simulink model "hybrid_model"  (R2021a)
settings: Solver=ode4  StartTime=0.0  StopTime=TMax  FixedStep=DT  MaxStep=DT  RelTol=1e-3  EnableMultiTasking=on
undefined symbols (not defined in the file or in its folder): OutList, strmatch
settings Model: Creator=bjonkman  LastModifiedBy=cam
settings SolverCC: AlgebraicLoopSolver=TrustRegion
settings DataIOCC: LimitDataPoints=on  SaveFormat=Array  SaveOutput=off  SaveTime=off  ReturnWorkspaceOutputs=off  SignalLoggingName=sigsOut
settings OptimizationCC: ExpressionDepthLimit=2147483647  LifeSpan=inf
settings DebuggingCC: SaveWithParameterizedLinksMsg=none  UnderspecifiedInitializationDetection=Classic  MergeDetectMultiDrivingBlocksExec=none  SignalResolutionControl=TryResolveAllWithWarning  InheritedTsInSrcMsg=none  MultiTaskDSMMsg=warning  MultiTaskCondExecSysMsg=none  FcnCallInpInsideContextMsg=warning  StateNameClashWarn=warning  SFUnexpectedBacktrackingDiag=warning  SFNoUnconditionalDefaultTransitionDiag=warning  SFExecutionAtInitializationDiag=none  SFMachineParentedDataDiag=warning  ArithmeticOperatorsInVariantConditions=warning
settings HardwareCC: ProdBitPerPointer=32  ProdBitPerSizeT=32  ProdBitPerPtrDiffT=32  ProdLargestAtomicFloat=None  ProdIntDivRoundTo=Undefined  ProdEndianess=Unspecified  ProdWordSize=32  ProdHWDeviceType=32-bit Generic  TargetBitPerLong=64  TargetBitPerPointer=64  TargetBitPerSizeT=64  TargetBitPerPtrDiffT=64  TargetLongLongMode=on  TargetIntDivRoundTo=Zero  TargetEndianess=LittleEndian  TargetWordSize=64  TargetHWDeviceType=MATLAB Host  ProdEqTarget=off
settings ModelReferenceCC: PropagateSignalLabelsOutOfModel=off
settings SFSimCC: SimUseLocalCustomCode=off  CustomCodeUndefinedFunction=UseInterfaceOnly
settings RTWCC: RTWUseLocalCustomCode=off
settings CodeAppCC: StateflowObjectComments=on
settings GRTTargetCC: TargetLangStandard=C89/C90 (ANSI)  CombineOutputUpdateFcns=off  GRTInterface=on
settings ConfigComp: CovMetricSettings=dw  CovSaveCumulativeToWorkspaceVar=on  CovSaveSingleToWorkspaceVar=on  CovExternalEMLEnable=off

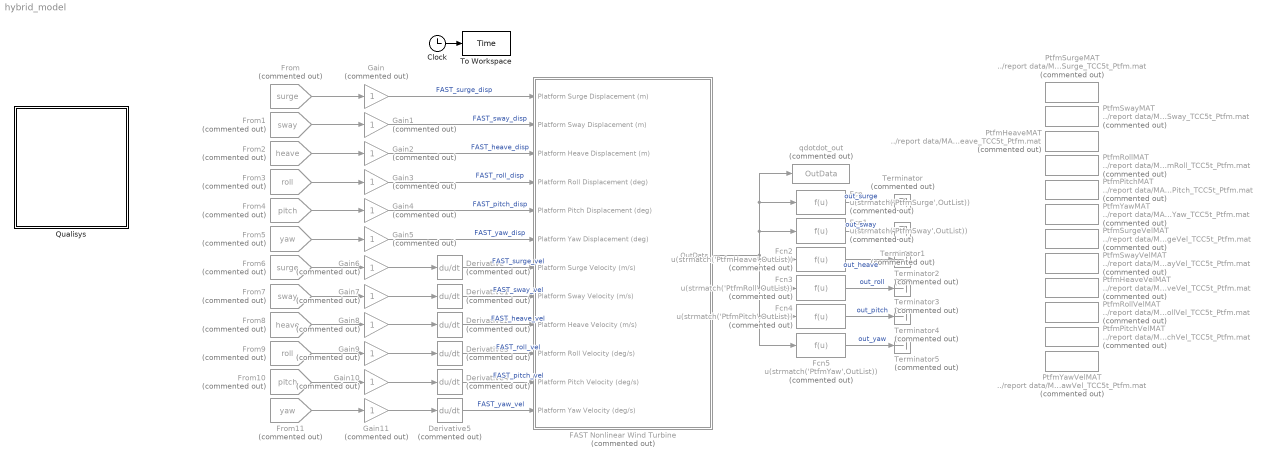
== system hybrid_model ==
  Clock : Clock
  Derivative{,1..5} (6 alike) : Derivative  Commented=on
  FAST Nonlinear Wind Turbine : Subsystem  Commented=on  mask(FAST Nonlinear Wind Turbine){}
      mask help: This block contains the FAST S-Function.
      mask init:
      | clear FAST_SFunc
  Fcn : Fcn  Commented=on  Expr=u(strmatch('PtfmSurge',OutList))
  Fcn1 : Fcn  Commented=on  Expr=u(strmatch('PtfmSway',OutList))
  Fcn2 : Fcn  Commented=on  Expr=u(strmatch('PtfmHeave',OutList))
  Fcn3 : Fcn  Commented=on  Expr=u(strmatch('PtfmRoll',OutList))
  Fcn4 : Fcn  Commented=on  Expr=u(strmatch('PtfmPitch',OutList))
  Fcn5 : Fcn  Commented=on  Expr=u(strmatch('PtfmYaw',OutList))
  From : From  Commented=on  GotoTag=surge  TagVisibility=global
  From1 : From  Commented=on  GotoTag=sway  TagVisibility=global
  From10 : From  Commented=on  GotoTag=pitch  TagVisibility=global
  From11 : From  Commented=on  GotoTag=yaw  TagVisibility=global
  From2 : From  Commented=on  GotoTag=heave  TagVisibility=global
  From3 : From  Commented=on  GotoTag=roll  TagVisibility=global
  From4 : From  Commented=on  GotoTag=pitch  TagVisibility=global
  From5 : From  Commented=on  GotoTag=yaw  TagVisibility=global
  From6 : From  Commented=on  GotoTag=surge  TagVisibility=global
  From7 : From  Commented=on  GotoTag=sway  TagVisibility=global
  From8 : From  Commented=on  GotoTag=heave  TagVisibility=global
  From9 : From  Commented=on  GotoTag=roll  TagVisibility=global
  Gain{,1..11} (12 alike) : Gain  Commented=on
  PtfmHeaveMAT : FromFile  Commented=on  FileName=../report data/MAT/PtfmHeave_TCC5t_Ptfm.mat
  PtfmHeaveVelMAT : FromFile  Commented=on  FileName=../report data/MAT/PtfmHeaveVel_TCC5t_Ptfm.mat
  PtfmPitchMAT : FromFile  Commented=on  FileName=../report data/MAT/PtfmPitch_TCC5t_Ptfm.mat
  PtfmPitchVelMAT : FromFile  Commented=on  FileName=../report data/MAT/PtfmPitchVel_TCC5t_Ptfm.mat
  PtfmRollMAT : FromFile  Commented=on  FileName=../report data/MAT/PtfmRoll_TCC5t_Ptfm.mat
  PtfmRollVelMAT : FromFile  Commented=on  FileName=../report data/MAT/PtfmRollVel_TCC5t_Ptfm.mat
  PtfmSurgeMAT : FromFile  Commented=on  FileName=../report data/MAT/PtfmSurge_TCC5t_Ptfm.mat
  PtfmSurgeVelMAT : FromFile  Commented=on  FileName=../report data/MAT/PtfmSurgeVel_TCC5t_Ptfm.mat
  PtfmSwayMAT : FromFile  Commented=on  FileName=../report data/MAT/PtfmSway_TCC5t_Ptfm.mat
  PtfmSwayVelMAT : FromFile  Commented=on  FileName=../report data/MAT/PtfmSwayVel_TCC5t_Ptfm.mat
  PtfmYawMAT : FromFile  Commented=on  FileName=../report data/MAT/PtfmYaw_TCC5t_Ptfm.mat
  PtfmYawVelMAT : FromFile  Commented=on  FileName=../report data/MAT/PtfmYawVel_TCC5t_Ptfm.mat
  Qualisys : Subsystem
  Terminator{,1..5} (6 alike) : Terminator  Commented=on
  To Workspace : ToWorkspace  VariableName=Time  SampleTime=-1
  qdotdot_out : ToWorkspace  Commented=on  VariableName=OutData  SampleTime=-1
  wires:
  Clock/1 -> To Workspace/1
  Gain/1 -> FAST Nonlinear Wind Turbine/1(Platform Surge Displacement (m))  "FAST_surge_disp"
  Gain5/1 -> FAST Nonlinear Wind Turbine/6(Platform Yaw Displacement (deg))  "FAST_yaw_disp"
  Gain4/1 -> FAST Nonlinear Wind Turbine/5(Platform Pitch Displacement (deg))  "FAST_pitch_disp"
  Gain3/1 -> FAST Nonlinear Wind Turbine/4(Platform Roll Displacement (deg))  "FAST_roll_disp"
  Gain2/1 -> FAST Nonlinear Wind Turbine/3(Platform Heave Displacement (m))  "FAST_heave_disp"
  From1/1 -> Gain1/1
  FAST Nonlinear Wind Turbine/1(OutData) -> qdotdot_out/1, Fcn/1, Fcn1/1, Fcn5/1, Fcn4/1, Fcn3/1, Fcn2/1
  Fcn/1 -> Terminator/1  "out_surge"
  Fcn1/1 -> Terminator1/1  "out_sway"
  Fcn5/1 -> Terminator5/1  "out_yaw"
  Fcn4/1 -> Terminator4/1  "out_pitch"
  Fcn3/1 -> Terminator3/1  "out_roll"
  Fcn2/1 -> Terminator2/1  "out_heave"
  Derivative1/1 -> FAST Nonlinear Wind Turbine/8(Platform Sway Velocity (m/s))  "FAST_sway_vel"
  Derivative3/1 -> FAST Nonlinear Wind Turbine/10(Platform Roll Velocity (deg/s))  "FAST_roll_vel"
  Derivative2/1 -> FAST Nonlinear Wind Turbine/9(Platform Heave Velocity (m/s))  "FAST_heave_vel"
  Derivative5/1 -> FAST Nonlinear Wind Turbine/12(Platform Yaw Velocity (deg/s))  "FAST_yaw_vel"
  Derivative4/1 -> FAST Nonlinear Wind Turbine/11(Platform Pitch Velocity (deg/s))  "FAST_pitch_vel"
  Derivative/1 -> FAST Nonlinear Wind Turbine/7(Platform Surge Velocity (m/s))  "FAST_surge_vel"
  From/1 -> Gain/1
  Gain1/1 -> FAST Nonlinear Wind Turbine/2(Platform Sway Displacement (m))  "FAST_sway_disp"
  From2/1 -> Gain2/1
  From3/1 -> Gain3/1
  From4/1 -> Gain4/1
  From5/1 -> Gain5/1
  From6/1 -> Gain6/1
  From11/1 -> Gain11/1
  From7/1 -> Gain7/1
  From8/1 -> Gain8/1
  From10/1 -> Gain10/1
  From9/1 -> Gain9/1
  Gain6/1 -> Derivative/1
  Gain7/1 -> Derivative1/1
  Gain8/1 -> Derivative2/1
  Gain9/1 -> Derivative3/1
  Gain10/1 -> Derivative4/1
  Gain11/1 -> Derivative5/1

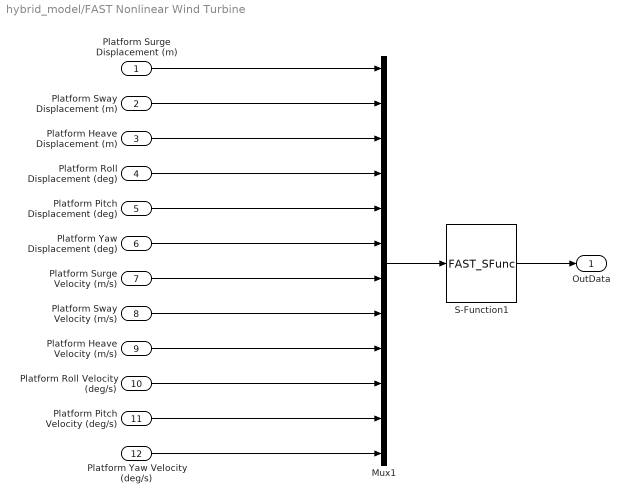
== system hybrid_model/FAST Nonlinear Wind Turbine ==
  Platform Surge Displacement (m) : Inport
  Platform Sway Displacement (m) : Inport  Port=2
  Platform Heave Displacement (m) : Inport  Port=3
  Platform Roll Displacement (deg) : Inport  Port=4
  Platform Pitch Displacement (deg) : Inport  Port=5
  Platform Yaw Displacement (deg) : Inport  Port=6
  Platform Surge Velocity (m/s) : Inport  Port=7
  Platform Sway Velocity (m/s) : Inport  Port=8
  Platform Heave Velocity (m/s) : Inport  Port=9
  Platform Roll Velocity (deg/s) : Inport  Port=10
  Platform Pitch Velocity (deg/s) : Inport  Port=11
  Platform Yaw Velocity (deg/s) : Inport  Port=12
  Mux1 : Mux  Inputs=12
  S-Function1 : S-Function  FunctionName=FAST_SFunc  Parameters=FAST_InputFileName, TMax, 0  SFunctionDeploymentMode=off  EnableBusSupport=off
  OutData : Outport
  wires:
  S-Function1/1 -> OutData/1
  Mux1/1 -> S-Function1/1
  Platform Surge Displacement (m)/1 -> Mux1/1
  Platform Sway Displacement (m)/1 -> Mux1/2
  Platform Heave Displacement (m)/1 -> Mux1/3
  Platform Roll Displacement (deg)/1 -> Mux1/4
  Platform Pitch Displacement (deg)/1 -> Mux1/5
  Platform Yaw Displacement (deg)/1 -> Mux1/6
  Platform Surge Velocity (m/s)/1 -> Mux1/7
  Platform Yaw Velocity (deg/s)/1 -> Mux1/12
  Platform Pitch Velocity (deg/s)/1 -> Mux1/11
  Platform Roll Velocity (deg/s)/1 -> Mux1/10
  Platform Heave Velocity (m/s)/1 -> Mux1/9
  Platform Sway Velocity (m/s)/1 -> Mux1/8

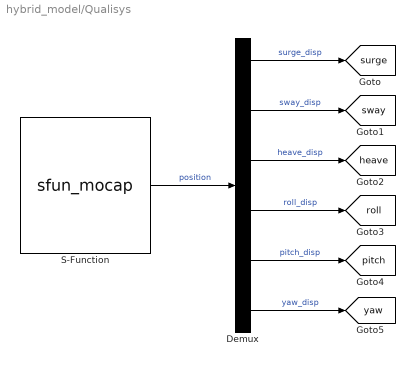
== system hybrid_model/Qualisys ==
  Demux : Demux  Outputs=6
  S-Function : S-Function  FunctionName=sfun_mocap  SFunctionDeploymentMode=off  EnableBusSupport=off
  tag scope: heave=global, pitch=global, roll=global, surge=global, sway=global, yaw=global
  wires:
  S-Function/1 -> Demux/1  "position"
  Demux/1 -> [surge]  "surge_disp"
  Demux/5 -> [pitch]  "pitch_disp"
  Demux/3 -> [heave]  "heave_disp"
  Demux/4 -> [roll]  "roll_disp"
  Demux/6 -> [yaw]  "yaw_disp"
  Demux/2 -> [sway]  "sway_disp"
